simulink model "untitled1"  (R2015b)
settings: Solver=VariableStepAuto  StartTime=0.0  StopTime=10.0  RelTol=1e-3
undefined symbols (not defined in the file): a, Ap, b, c, Csfl, Csfr, Csrl, Csrr, d, Ixx, Iyy, Ksfl, Ksfr, Ksrl, Ksrr, M, S
settings Model: Creator=Guest  LastModifiedBy=Guest

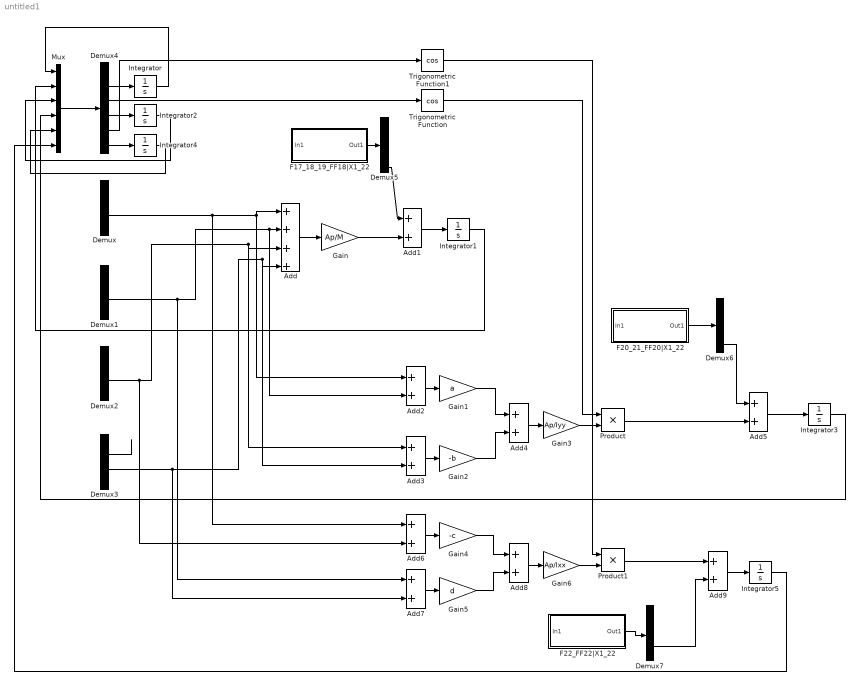
== system untitled1 ==
  Add : Sum  Inputs=4
  Add{1..9} (9 alike) : Sum  Inputs=2
  Demux{,1..3,5} (5 alike) : Demux
  Demux4 : Demux  Outputs=6
  Demux6 : Demux  Outputs=3
  Demux7 : Demux  Outputs=2
  F17_18_19_FF18|X1_22 : Subsystem  TreatAsAtomicUnit=on
  "F20_21_FF20|X1_22 " : Subsystem  TreatAsAtomicUnit=on
  F22_FF22|X1_22 : Subsystem  TreatAsAtomicUnit=on
  Gain : Gain  Gain=Ap/M
  Gain1 : Gain  Gain=a
  Gain2 : Gain  Gain=-b
  Gain3 : Gain  Gain=Ap/Iyy
  Gain4 : Gain  Gain=-c
  Gain5 : Gain  Gain=d
  Gain6 : Gain  Gain=Ap/Ixx
  Integrator{,1..5} (6 alike) : Integrator
  Mux : Mux  Inputs=6
  Product : Product
  Product1 : Product
  Trigonometric Function : Trigonometry  Operator=cos
  Trigonometric Function1 : Trigonometry  Operator=cos
  wires:
  Demux3/2 -> ?
  Mux/1 -> Demux4/1
  Demux4/2 -> Integrator/1
  Integrator/1 -> Mux/1
  Demux/3 -> Add6/1, Add2/1, Add/1
  Demux1/3 -> Add7/1, Add2/2, Add/2
  Demux2/3 -> Add6/2, Add3/1, Add/3
  Demux3/3 -> Add7/2, Add3/2, Add/4
  Add/1 -> Gain/1
  F17_18_19_FF18|X1_22/1(Out1) -> Demux5/1
  Gain/1 -> Add1/2
  Demux5/4 -> Add1/1
  Add1/1 -> Integrator1/1
  Integrator1/1 -> Mux/2
  Demux4/4 -> Integrator2/1
  Integrator2/1 -> Mux/3
  Add2/1 -> Gain1/1
  Add3/1 -> Gain2/1
  Gain1/1 -> Add4/1
  Gain2/1 -> Add4/2
  Add4/1 -> Gain3/1
  Demux4/3 -> Trigonometric Function/1
  Gain3/1 -> Product/2
  Trigonometric Function/1 -> Product/1
  "F20_21_FF20|X1_22 "/1(Out1) -> Demux6/1
  Product/1 -> Add5/2
  Demux6/3 -> Add5/1
  Add5/1 -> Integrator3/1
  Integrator3/1 -> Mux/4
  Demux4/6 -> Integrator4/1
  Integrator4/1 -> Mux/5
  Add6/1 -> Gain4/1
  Add7/1 -> Gain5/1
  Gain4/1 -> Add8/1
  Gain5/1 -> Add8/2
  Add8/1 -> Gain6/1
  Gain6/1 -> Product1/2
  Demux4/5 -> Trigonometric Function1/1
  Trigonometric Function1/1 -> Product1/1
  F22_FF22|X1_22/1(Out1) -> Demux7/1
  Demux7/2 -> Add9/2
  Product1/1 -> Add9/1
  Add9/1 -> Integrator5/1
  Integrator5/1 -> Mux/6

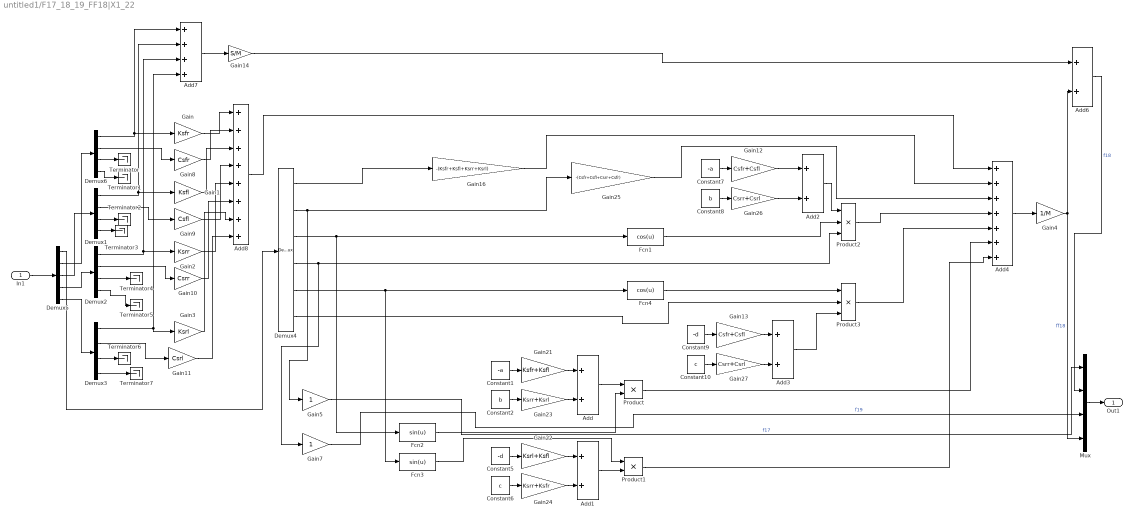
== system untitled1/F17_18_19_FF18|X1_22 ==
  In1 : Inport
  Add{,1..3,6} (5 alike) : Sum
  Add4 : Sum  Inputs=+++++++
  Add7 : Sum  Inputs=++++
  Add8 : Sum  Inputs=++++++++
  Constant1 : Constant  Value=-a
  Constant10 : Constant  Value=c
  Constant2 : Constant  Value=b
  Constant5 : Constant  Value=-d
  Constant6 : Constant  Value=c
  Constant7 : Constant  Value=-a
  Constant8 : Constant  Value=b
  Constant9 : Constant  Value=-d
  Demux{1..3,6} (4 alike) : Demux
  Demux4 : Demux  Outputs=6
  Demux5 : Demux  Outputs=5
  Fcn1 : Fcn  Expr=cos(u)
  Fcn2 : Fcn  Expr=sin(u)
  Fcn3 : Fcn  Expr=sin(u)
  Fcn4 : Fcn  Expr=cos(u)
  Gain : Gain  Gain=Ksfr
  Gain1 : Gain  Gain=Ksfl
  Gain10 : Gain  Gain=Csrr
  Gain11 : Gain  Gain=Csrl
  Gain12 : Gain  Gain=Csfr+Csfl
  Gain13 : Gain  Gain=Csfr+Csfl
  Gain14 : Gain  Gain=S/M
  Gain16 : Gain  Gain=-(Ksfr+Ksfl+Ksrr+Ksrl)
  Gain2 : Gain  Gain=Ksrr
  Gain21 : Gain  Gain=Ksfr+Ksfl
  Gain22 : Gain  Gain=Ksrl+Ksfl
  Gain23 : Gain  Gain=Ksrr+Ksrl
  Gain24 : Gain  Gain=Ksrr+Ksfr
  Gain25 : Gain  Gain=-(Csfr+Csfl+Csrr+Csfr)
  Gain26 : Gain  Gain=Csrr+Csrl
  Gain27 : Gain  Gain=Csrr+Csrl
  Gain3 : Gain  Gain=Ksrl
  Gain4 : Gain  Gain=1/M
  Gain5 : Gain
  Gain7 : Gain
  Gain8 : Gain  Gain=Csfr
  Gain9 : Gain  Gain=Csfl
  Mux : Mux
  Product : Product
  Product1 : Product
  Product2 : Product  Inputs=3
  Product3 : Product  Inputs=3
  Terminator{,1..7} (8 alike) : Terminator
  Out1 : Outport
  wires:
  Demux6/1 -> Add7/1, Gain/1
  Demux1/1 -> Gain1/1, Add7/2
  Demux2/1 -> Gain2/1, Add7/3
  Demux3/1 -> Gain3/1, Add7/4
  Demux4/1 -> Gain16/1
  Demux4/3 -> Fcn2/1, Fcn1/1
  Gain21/1 -> Add/1
  Constant1/1 -> Gain21/1
  Gain23/1 -> Add/2
  Constant2/1 -> Gain23/1
  Add/1 -> Product/1
  Fcn2/1 -> Product/2
  Demux4/5 -> Fcn3/1, Fcn4/1
  Gain22/1 -> Add1/1
  Gain24/1 -> Add1/2
  Constant5/1 -> Gain22/1
  Constant6/1 -> Gain24/1
  Add1/1 -> Product1/2
  Fcn3/1 -> Product1/1
  Demux4/2 -> Gain5/1, Gain25/1
  Demux4/4 -> Gain7/1, Product2/3
  Fcn1/1 -> Product2/2
  Gain12/1 -> Add2/1
  Constant7/1 -> Gain12/1
  Gain26/1 -> Add2/2
  Constant8/1 -> Gain26/1
  Add2/1 -> Product2/1
  Gain13/1 -> Add3/1
  Constant9/1 -> Gain13/1
  Gain27/1 -> Add3/2
  Constant10/1 -> Gain27/1
  Fcn4/1 -> Product3/1
  Demux4/6 -> Product3/2
  Add3/1 -> Product3/3
  Product/1 -> Add4/6
  Product1/1 -> Add4/7
  Add4/1 -> Gain4/1
  Gain14/1 -> Add6/1
  Gain4/1 -> Add6/2, Mux/4  "ff18"
  Add6/1 -> Mux/2  "f18"
  Gain5/1 -> Mux/1  "f17"
  Gain7/1 -> Mux/3  "f19"
  Demux6/2 -> Gain8/1
  Demux1/2 -> Gain9/1
  Demux2/2 -> Gain10/1
  Demux3/2 -> Gain11/1
  Add7/1 -> Gain14/1
  Gain/1 -> Add8/1
  Gain8/1 -> Add8/2
  Gain1/1 -> Add8/3
  Gain9/1 -> Add8/4
  Gain2/1 -> Add8/5
  Gain10/1 -> Add8/6
  Gain3/1 -> Add8/7
  Gain11/1 -> Add8/8
  Product3/1 -> Add4/5
  Product2/1 -> Add4/4
  Gain25/1 -> Add4/3
  Gain16/1 -> Add4/2
  Add8/1 -> Add4/1
  Demux6/3 -> Terminator/1
  Demux6/4 -> Terminator1/1
  Demux1/3 -> Terminator2/1
  Demux1/4 -> Terminator3/1
  Demux2/3 -> Terminator4/1
  Demux2/4 -> Terminator5/1
  Demux3/3 -> Terminator6/1
  Demux3/4 -> Terminator7/1
  Demux5/2 -> Demux6/1
  Demux5/3 -> Demux1/1
  Demux5/4 -> Demux2/1
  Demux5/5 -> Demux3/1
  In1/1 -> Demux5/1
  Mux/1 -> Out1/1
  Demux5/1 -> Demux4/1

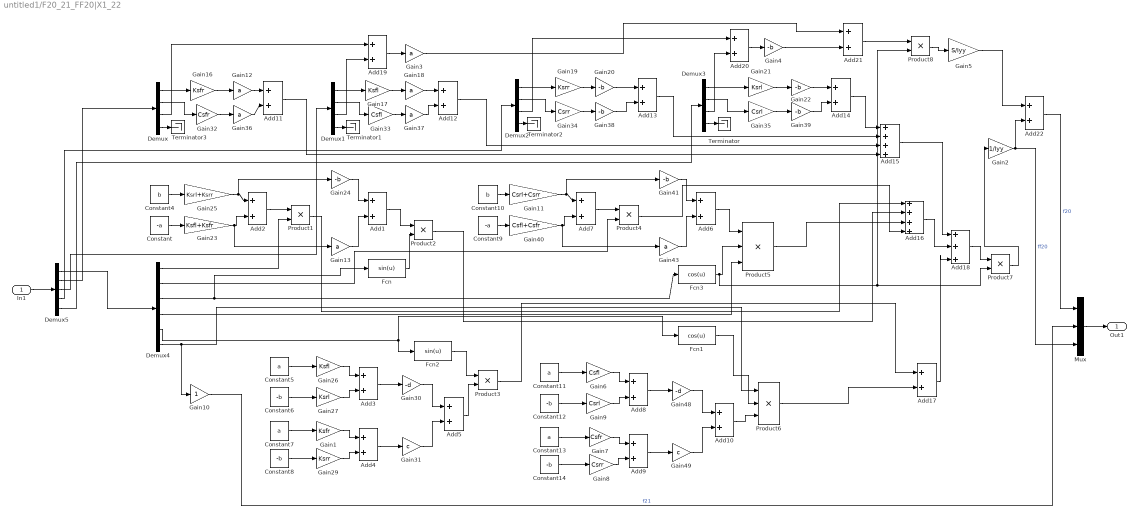
== system untitled1/F20_21_FF20|X1_22  ==
  In1 : Inport
  Add{1..14,17,19..22} (19 alike) : Sum
  Add15 : Sum  Inputs=++++
  Add16 : Sum  Inputs=++++
  Add18 : Sum  Inputs=+++
  Constant : Constant  Value=-a
  Constant10 : Constant  Value=b
  Constant{5,7,11,13} (4 alike) : Constant  Value=a
  Constant{6,8,12,14} (4 alike) : Constant  Value=-b
  Constant4 : Constant  Value=b
  Constant9 : Constant  Value=-a
  Demux{,1..3} (4 alike) : Demux
  Demux4 : Demux  Outputs=6
  Demux5 : Demux  Outputs=5
  Fcn : Fcn  Expr=sin(u)
  Fcn1 : Fcn  Expr=cos(u)
  Fcn2 : Fcn  Expr=sin(u)
  Fcn3 : Fcn  Expr=cos(u)
  Gain1 : Gain  Gain=Ksfr
  Gain10 : Gain
  Gain11 : Gain  Gain=Csrl+Csrr
  Gain{3,12..13,18,36..37,43} (7 alike) : Gain  Gain=a
  Gain16 : Gain  Gain=Ksfr
  Gain17 : Gain  Gain=Ksfl
  Gain19 : Gain  Gain=Ksrr
  Gain2 : Gain  Gain=1/Iyy
  Gain{4,20,22,24,38..39,41} (7 alike) : Gain  Gain=-b
  Gain21 : Gain  Gain=Ksrl
  Gain23 : Gain  Gain=Ksfl+Ksfr
  Gain25 : Gain  Gain=Ksrl+Ksrr
  Gain26 : Gain  Gain=Ksfl
  Gain27 : Gain  Gain=Ksrl
  Gain29 : Gain  Gain=Ksrr
  Gain30 : Gain  Gain=-d
  Gain31 : Gain  Gain=c
  Gain32 : Gain  Gain=Csfr
  Gain33 : Gain  Gain=Csfl
  Gain34 : Gain  Gain=Csrr
  Gain35 : Gain  Gain=Csrl
  Gain40 : Gain  Gain=Csfl+Csfr
  Gain48 : Gain  Gain=-d
  Gain49 : Gain  Gain=c
  Gain5 : Gain  Gain=S/Iyy
  Gain6 : Gain  Gain=Csfl
  Gain7 : Gain  Gain=Csfr
  Gain8 : Gain  Gain=Csrr
  Gain9 : Gain  Gain=Csrl
  Mux : Mux  Inputs=3
  Product{1..4,7..8} (6 alike) : Product
  Product5 : Product  Inputs=3
  Product6 : Product  Inputs=3
  Terminator{,1..3} (4 alike) : Terminator
  Out1 : Outport
  wires:
  Demux/1 -> Gain16/1
  Gain16/1 -> Gain12/1
  Demux1/1 -> Gain17/1
  Gain17/1 -> Gain18/1
  Demux2/1 -> Gain19/1
  Gain19/1 -> Gain20/1
  Demux3/1 -> Gain21/1
  Gain21/1 -> Gain22/1
  Constant/1 -> Gain23/1
  Constant4/1 -> Gain25/1
  Gain23/1 -> Gain13/1, Add2/2
  Gain25/1 -> Gain24/1, Add2/1
  Add2/1 -> Product1/1
  Demux4/1 -> Product1/2
  Gain24/1 -> Add1/1
  Gain13/1 -> Add1/2
  Constant5/1 -> Gain26/1
  Constant6/1 -> Gain27/1
  Gain26/1 -> Add3/1
  Gain27/1 -> Add3/2
  Constant8/1 -> Gain29/1
  Constant7/1 -> Gain1/1
  Gain1/1 -> Add4/1
  Gain29/1 -> Add4/2
  Add3/1 -> Gain30/1
  Add4/1 -> Gain31/1
  Demux4/3 -> Fcn3/1, Fcn/1
  Add1/1 -> Product2/1
  Fcn/1 -> Product2/2
  Demux4/5 -> Fcn1/1, Fcn2/1
  Gain30/1 -> Add5/1
  Gain31/1 -> Add5/2
  Add5/1 -> Product3/2
  Fcn2/1 -> Product3/1
  Demux/2 -> Gain32/1
  Demux1/2 -> Gain33/1
  Demux2/2 -> Gain34/1
  Demux3/2 -> Gain35/1
  Gain32/1 -> Gain36/1
  Gain33/1 -> Gain37/1
  Gain34/1 -> Gain38/1
  Gain35/1 -> Gain39/1
  Constant10/1 -> Gain11/1
  Gain40/1 -> Gain43/1, Add7/2
  Gain11/1 -> Add7/1, Gain41/1
  Add7/1 -> Product4/1
  Demux4/2 -> Product4/2
  Gain41/1 -> Add6/1
  Gain43/1 -> Add6/2
  Add6/1 -> Product5/1
  Constant9/1 -> Gain40/1
  Fcn3/1 -> Product8/2, Product7/2, Product5/2
  Demux4/4 -> Product5/3
  Constant11/1 -> Gain6/1
  Constant12/1 -> Gain9/1
  Gain6/1 -> Add8/1
  Gain9/1 -> Add8/2
  Constant14/1 -> Gain8/1
  Constant13/1 -> Gain7/1
  Gain7/1 -> Add9/1
  Add8/1 -> Gain48/1
  Add9/1 -> Gain49/1
  Gain48/1 -> Add10/1
  Gain49/1 -> Add10/2
  Add10/1 -> Product6/3
  Fcn1/1 -> Product6/2
  Gain8/1 -> Add9/2
  Demux4/6 -> Gain10/1, Product6/1
  Gain12/1 -> Add11/1
  Gain36/1 -> Add11/2
  Gain18/1 -> Add12/1
  Gain37/1 -> Add12/2
  Gain20/1 -> Add13/1
  Gain38/1 -> Add13/2
  Gain22/1 -> Add14/1
  Gain39/1 -> Add14/2
  Add14/1 -> Add15/1
  Add13/1 -> Add15/2
  Add12/1 -> Add15/3
  Add11/1 -> Add15/4
  Product1/1 -> Add16/1
  Product2/1 -> Add16/2
  Product5/1 -> Add16/3
  Product4/1 -> Add16/4
  Product3/1 -> Add17/1
  Product6/1 -> Add17/2
  Add15/1 -> Add18/1
  Add17/1 -> Add18/3
  Add16/1 -> Add18/2
  Add18/1 -> Product7/1
  Product7/1 -> Gain2/1
  Demux/3 -> Add19/1
  Demux1/3 -> Add19/2
  Add19/1 -> Gain3/1
  Demux2/3 -> Add20/1
  Demux3/3 -> Add20/2
  Add20/1 -> Gain4/1
  Gain4/1 -> Add21/2
  Gain3/1 -> Add21/1
  Add21/1 -> Product8/1
  Product8/1 -> Gain5/1
  Gain5/1 -> Add22/1
  Gain2/1 -> Mux/3, Add22/2  "ff20"
  Gain10/1 -> Mux/2  "f21"
  Add22/1 -> Mux/1  "f20"
  Demux1/4 -> Terminator1/1
  Demux2/4 -> Terminator2/1
  Demux3/4 -> Terminator/1
  Demux/4 -> Terminator3/1
  Demux5/1 -> Demux4/1
  Demux5/2 -> Demux/1
  Demux5/3 -> Demux1/1
  Demux5/4 -> Demux2/1
  Demux5/5 -> Demux3/1
  In1/1 -> Demux5/1
  Mux/1 -> Out1/1

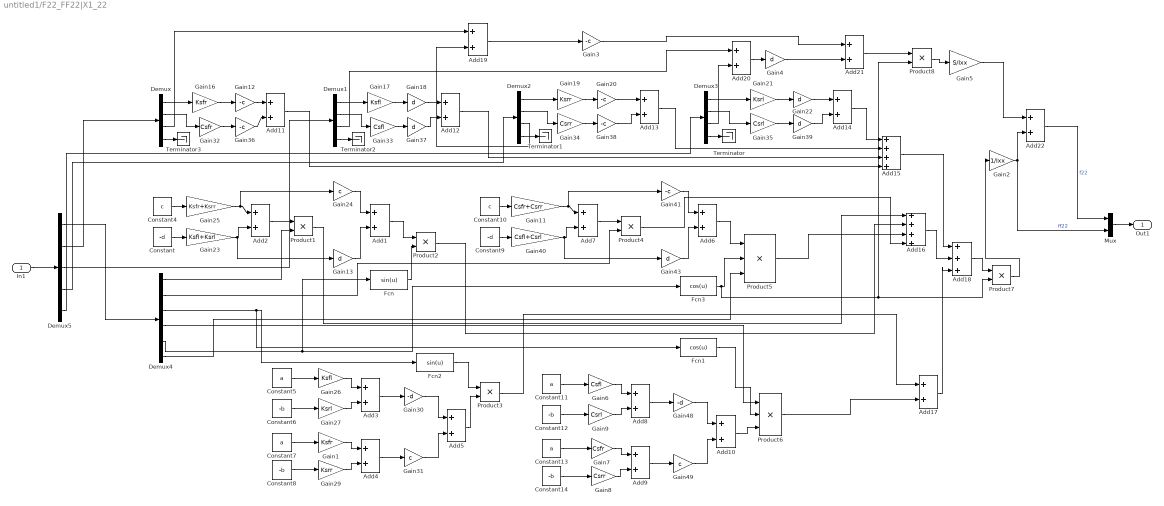
== system untitled1/F22_FF22|X1_22 ==
  In1 : Inport
  Add{1..14,17,19..22} (19 alike) : Sum
  Add15 : Sum  Inputs=++++
  Add16 : Sum  Inputs=++++
  Add18 : Sum  Inputs=+++
  Constant : Constant  Value=-d
  Constant10 : Constant  Value=c
  Constant{5,7,11,13} (4 alike) : Constant  Value=a
  Constant{6,8,12,14} (4 alike) : Constant  Value=-b
  Constant4 : Constant  Value=c
  Constant9 : Constant  Value=-d
  Demux{,1..3} (4 alike) : Demux
  Demux4 : Demux  Outputs=6
  Demux5 : Demux  Outputs=5
  Fcn : Fcn  Expr=sin(u)
  Fcn1 : Fcn  Expr=cos(u)
  Fcn2 : Fcn  Expr=sin(u)
  Fcn3 : Fcn  Expr=cos(u)
  Gain1 : Gain  Gain=Ksfr
  Gain11 : Gain  Gain=Csfr+Csrr
  Gain{3,12,20,36,38,41} (6 alike) : Gain  Gain=-c
  Gain{4,13,18,22,37,39,43} (7 alike) : Gain  Gain=d
  Gain16 : Gain  Gain=Ksfr
  Gain17 : Gain  Gain=Ksfl
  Gain19 : Gain  Gain=Ksrr
  Gain2 : Gain  Gain=1/Ixx
  Gain21 : Gain  Gain=Ksrl
  Gain23 : Gain  Gain=Ksfl+Ksrl
  Gain24 : Gain  Gain=c
  Gain25 : Gain  Gain=Ksfr+Ksrr
  Gain26 : Gain  Gain=Ksfl
  Gain27 : Gain  Gain=Ksrl
  Gain29 : Gain  Gain=Ksrr
  Gain30 : Gain  Gain=-d
  Gain31 : Gain  Gain=c
  Gain32 : Gain  Gain=Csfr
  Gain33 : Gain  Gain=Csfl
  Gain34 : Gain  Gain=Csrr
  Gain35 : Gain  Gain=Csrl
  Gain40 : Gain  Gain=Csfl+Csrl
  Gain48 : Gain  Gain=-d
  Gain49 : Gain  Gain=c
  Gain5 : Gain  Gain=S/Ixx
  Gain6 : Gain  Gain=Csfl
  Gain7 : Gain  Gain=Csfr
  Gain8 : Gain  Gain=Csrr
  Gain9 : Gain  Gain=Csrl
  Mux : Mux  Inputs=2
  Product{1..4,7..8} (6 alike) : Product
  Product5 : Product  Inputs=3
  Product6 : Product  Inputs=3
  Terminator{,1..3} (4 alike) : Terminator
  Out1 : Outport
  wires:
  Demux/1 -> Gain16/1
  Gain16/1 -> Gain12/1
  Demux1/1 -> Gain17/1
  Gain17/1 -> Gain18/1
  Demux2/1 -> Gain19/1
  Gain19/1 -> Gain20/1
  Demux3/1 -> Gain21/1
  Gain21/1 -> Gain22/1
  Constant/1 -> Gain23/1
  Constant4/1 -> Gain25/1
  Gain23/1 -> Gain13/1, Add2/2
  Gain25/1 -> Gain24/1, Add2/1
  Add2/1 -> Product1/1
  Demux4/1 -> Product1/2
  Gain24/1 -> Add1/1
  Gain13/1 -> Add1/2
  Constant5/1 -> Gain26/1
  Constant6/1 -> Gain27/1
  Gain26/1 -> Add3/1
  Gain27/1 -> Add3/2
  Constant8/1 -> Gain29/1
  Constant7/1 -> Gain1/1
  Gain1/1 -> Add4/1
  Gain29/1 -> Add4/2
  Add3/1 -> Gain30/1
  Add4/1 -> Gain31/1
  Demux4/3 -> Fcn1/1, Fcn2/1
  Add1/1 -> Product2/1
  Fcn/1 -> Product2/2
  Demux4/5 -> Fcn/1, Fcn3/1
  Gain30/1 -> Add5/1
  Gain31/1 -> Add5/2
  Add5/1 -> Product3/2
  Fcn2/1 -> Product3/1
  Demux/2 -> Gain32/1
  Demux1/2 -> Gain33/1
  Demux2/2 -> Gain34/1
  Demux3/2 -> Gain35/1
  Gain32/1 -> Gain36/1
  Gain33/1 -> Gain37/1
  Gain34/1 -> Gain38/1
  Gain35/1 -> Gain39/1
  Constant10/1 -> Gain11/1
  Gain40/1 -> Gain43/1, Add7/2
  Gain11/1 -> Add7/1, Gain41/1
  Add7/1 -> Product4/1
  Demux4/2 -> Product4/2
  Gain41/1 -> Add6/1
  Gain43/1 -> Add6/2
  Add6/1 -> Product5/1
  Constant9/1 -> Gain40/1
  Fcn3/1 -> Product8/2, Product7/2, Product5/2
  Constant11/1 -> Gain6/1
  Constant12/1 -> Gain9/1
  Gain6/1 -> Add8/1
  Gain9/1 -> Add8/2
  Constant14/1 -> Gain8/1
  Constant13/1 -> Gain7/1
  Gain7/1 -> Add9/1
  Add8/1 -> Gain48/1
  Add9/1 -> Gain49/1
  Gain48/1 -> Add10/1
  Gain49/1 -> Add10/2
  Add10/1 -> Product6/3
  Fcn1/1 -> Product6/2
  Gain8/1 -> Add9/2
  Demux4/6 -> Product5/3
  Gain12/1 -> Add11/1
  Gain36/1 -> Add11/2
  Gain18/1 -> Add12/1
  Gain37/1 -> Add12/2
  Gain20/1 -> Add13/1
  Gain38/1 -> Add13/2
  Gain22/1 -> Add14/1
  Gain39/1 -> Add14/2
  Add14/1 -> Add15/1
  Add13/1 -> Add15/2
  Add12/1 -> Add15/3
  Add11/1 -> Add15/4
  Product1/1 -> Add16/1
  Product2/1 -> Add16/2
  Product5/1 -> Add16/3
  Product4/1 -> Add16/4
  Product3/1 -> Add17/1
  Product6/1 -> Add17/2
  Add15/1 -> Add18/1
  Add17/1 -> Add18/3
  Add16/1 -> Add18/2
  Add18/1 -> Product7/1
  Product7/1 -> Gain2/1
  Demux/3 -> Add19/1
  Add19/1 -> Gain3/1
  Add20/1 -> Gain4/1
  Gain4/1 -> Add21/2
  Gain3/1 -> Add21/1
  Add21/1 -> Product8/1
  Product8/1 -> Gain5/1
  Gain5/1 -> Add22/1
  Gain2/1 -> Add22/2, Mux/2  "ff22"
  Add22/1 -> Mux/1  "f22"
  Demux4/4 -> Product6/1
  Demux2/3 -> Add19/2
  Demux1/3 -> Add20/1
  Demux3/3 -> Add20/2
  Demux5/1 -> Demux4/1
  Demux5/2 -> Demux/1
  Demux5/3 -> Demux1/1
  Demux5/4 -> Demux2/1
  Demux5/5 -> Demux3/1
  Demux3/4 -> Terminator/1
  Demux2/4 -> Terminator1/1
  Demux1/4 -> Terminator2/1
  Demux/4 -> Terminator3/1
  In1/1 -> Demux5/1
  Mux/1 -> Out1/1
